simulink model "PM_motor"  (R2024a)
settings: Solver=VariableStepAuto  StartTime=0.0  StopTime=10.0  RelTol=1e-3
values from neighbouring files (symbols this model uses):
  Dm = 4.49e-4    (= 0.000449)    [parameter.m]
  J = 1.075    [parameter.m]
  Kv = 0.227    [parameter.m]
  La = 0.235e-3    (= 0.000235)    [parameter.m]
  Ra = 0.62    [parameter.m]
  Tm = 1.08    [parameter.m]
settings Model: Creator=Yoru  LastModifiedBy=Yoru

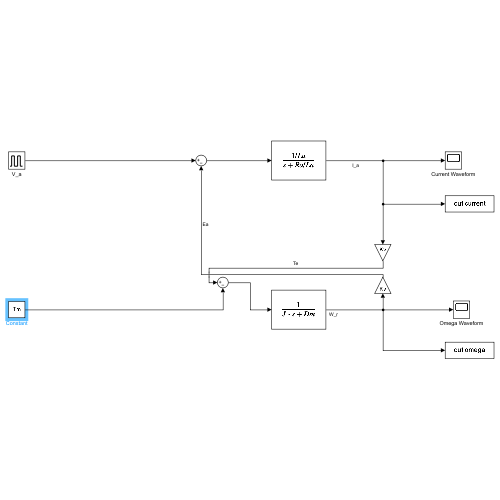
[thumbnail: Simulink's stored preview of the top-level diagram]
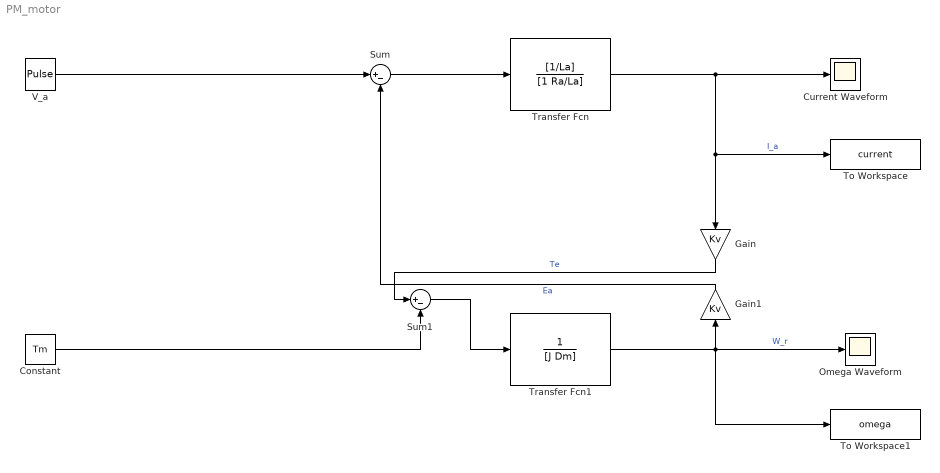
== system PM_motor ==
  Constant : Constant  Value=Tm
  Current Waveform : Scope
  Gain : Gain  Gain=Kv
  Gain1 : Gain  Gain=Kv
  Omega Waveform : Scope
  Sum : Sum  Inputs=|+-
  Sum1 : Sum  Inputs=|+-
  To Workspace : ToWorkspace  VariableName=current  SaveFormat=Timeseries  SampleTime=-1
  To Workspace1 : ToWorkspace  VariableName=omega  SaveFormat=Timeseries  SampleTime=-1
  Transfer Fcn : TransferFcn  Numerator=[1/La]  Denominator=[1 Ra/La]
  Transfer Fcn1 : TransferFcn  Denominator=[J Dm]
  V_a : DiscretePulseGenerator  PulseType=Time based  Amplitude=50  Period=1/10000  PulseWidth=90
  wires:
  V_a/1 -> Sum/1
  Sum/1 -> Transfer Fcn/1
  Transfer Fcn/1 -> Gain/1, To Workspace/1, Current Waveform/1  "I_a"
  Gain/1 -> Sum1/1  "Te"
  Constant/1 -> Sum1/2
  Sum1/1 -> Transfer Fcn1/1
  Transfer Fcn1/1 -> Omega Waveform/1, To Workspace1/1, Gain1/1  "W_r"
  Gain1/1 -> Sum/2  "Ea"
